simulink model "ex1"  (R2019a)
settings: Solver=VariableStepAuto  StartTime=0.0  StopTime=10  RelTol=1e-3
libraries: fuzblock x1, simulink x1
settings Model: Creator=maria  LastModifiedBy=maria

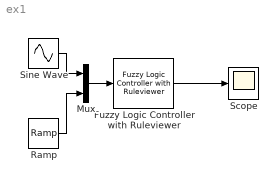
== system ex1 ==
  Fuzzy Logic Controller with Ruleviewer : fuzblock/Fuzzy Logic  Controller  with Ruleviewer  fismatrix=ex1  Ts=1
  Mux : Mux  Inputs=2
  Ramp : simulink/Sources/Ramp  slope=10  start=0  InitialOutput=0
  Scope : Scope
  Sine Wave : Sin  Amplitude=7  Bias=7  SampleTime=0
  wires:
  Mux/1 -> Fuzzy Logic Controller with Ruleviewer/1
  Ramp/1 -> Mux/2
  Sine Wave/1 -> Mux/1
  Fuzzy Logic Controller with Ruleviewer/1 -> Scope/1
